simulink model "gm_smartCart3"  (R2016a)
settings: Solver=FixedStepDiscrete  StartTime=0.0  StopTime=600000  FixedStep=1  RelTol=1e-3
libraries: simulink x56, hdlsllib x28
(part 2 of 2)

== system gm_smartCart3/head/Reciver/Unit Delay Enabled Resettable9 ==
  data_in : Inport
  Enb : Inport  Port=2
  Reset : Inport  Port=3
  Const_Zero : Constant  Value=0  OutDataTypeStr=boolean
  Initial_Condition : Constant  Value=0.0  OutDataTypeStr=Inherit: Inherit via back propagation
  OR : Logic  Operator=OR
  delay_down : UnitDelay  SampleTime=-1
  delay_up : UnitDelay  InitialCondition=1  SampleTime=-1
  switch0 : Switch  SaturateOnIntegerOverflow=on  InputSameDT=on
  switch1 : Switch  SaturateOnIntegerOverflow=on  InputSameDT=on
  switch2 : Switch  SaturateOnIntegerOverflow=on  InputSameDT=on
  data_out : Outport
  wires:
  data_in/1 -> switch0/1
  Enb/1 -> switch0/2
  switch2/1 -> switch0/3, data_out/1
  Initial_Condition/1 -> switch1/1, switch2/1
  Reset/1 -> switch1/2, OR/1
  switch0/1 -> switch1/3
  Const_Zero/1 -> delay_up/1
  switch1/1 -> delay_down/1
  delay_up/1 -> OR/2
  OR/1 -> switch2/2
  delay_down/1 -> switch2/3
